simulink model "PV_Microgrid_700V_avg"  (R2025b)
settings: Solver=ode1  StartTime=0.0  StopTime=86400  FixedStep=10  RelTol=1e-3
settings Model: Creator=PC  LastModifiedBy=PC
settings DataIOCC: SaveOutput=off

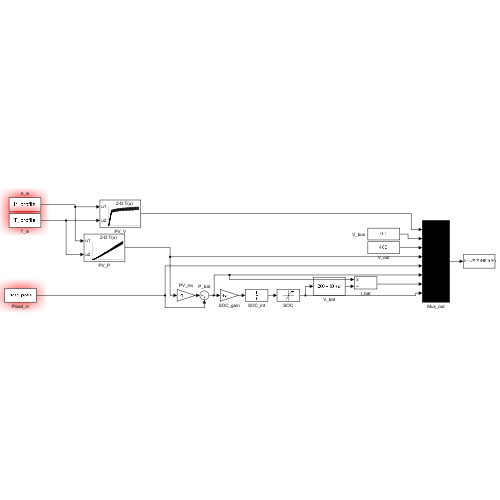
[thumbnail: Simulink's stored preview of the top-level diagram]
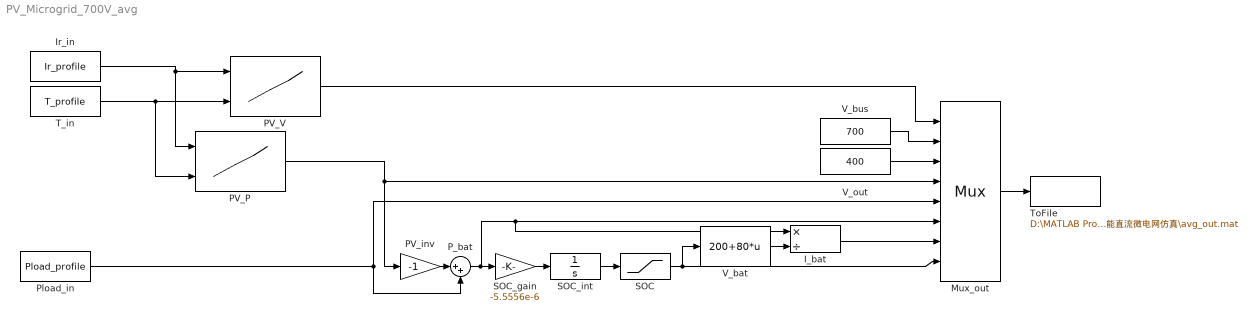
== system PV_Microgrid_700V_avg ==
  I_bat : Product  Inputs=*/
  Ir_in : FromWorkspace  VariableName=Ir_profile
  Mux_out : Mux  Inputs=8
  PV_P : Lookup_n-D  BreakpointsForDimension1=[0 100 200 300 400 500 600 700 800 900 1000]  BreakpointsForDimension2=[0 5 10 15 20 25 30 35 40 45]  Table=[0 0 0 0 0 0 0 0 0 0;479.267095176164 488.039274912844 496.8285763303 505.608509088825 514.379424979519 523.141658967104 531.90233605034 540.692996371929 549.47501520693 558.248690944814;1018.21000734054 1036.85645891559 1055.5023280483 1074.14764364788 1092.79243274262 1111.43672063028 1130.08053101432 1148.72388612752 1167.3668068442 1186.0093127824;1579.87273292352 1608.8143235643 1637.75152510228 1666.6845890358 1695.61374804727 1724.5392177273 1753.46119811304 1782.37987506345 1811.29542149157 1840.20799847052;2156.32163170459 2195.74523582645 2235.22493461024 2274.75056667442 2314.25580095053 2353.74186007896 2393.20987150242 2432.66087650542 2472.0958382476 2511.53595844375;2743.78589342684 2793.95276398475 2844.12262758078 2894.4417589686 2944.71315643147 2994.93984938429 3045.12461881785 3095.27002203532 3145.56779511549 3195.84887401155;3339.80841763825 3401.0911647803 3462.29044403554 3523.40716510524 3584.44687504203 3645.63503632356 3706.85652888916 3767.9997110104 3829.06951767878 3890.17475168714;3943.29173429922 4015.63363707419 4087.88520702704 4160.00939463728 4232.09113239226 4304.43299619547 4376.64909213525 4448.74777953302 4520.91939000649 4593.22084659552;4553.2053983687 4636.35277435902 4719.91035209304 4803.3036431147 4886.5208951813 4969.9265274586 5053.37839561389 5136.65963703153 5219.92730243945 5303.43282420516;5168.34686101416 5263.06947489515 5357.54448836249 5452.19614061513 5546.92870552013 5641.42542216233 5736.04537858514 5830.78693606171 5925.30333515889 6019.89458080095;5788.50808270469 5894.26936043688 6000.38379566756 6106.41353464746 6212.14007287575 6318.33198029437 6424.31326681351 6530.04226172463 6636.27038133268 6742.20810452584]  InternalRulePriority=Speed  RndMeth=Simplest
      settings: InputPortMap=u0,u1
  PV_V : Lookup_n-D  BreakpointsForDimension1=[0 100 200 300 400 500 600 700 800 900 1000]  BreakpointsForDimension2=[0 5 10 15 20 25 30 35 40 45]  Table=[0 0 0 0 0 0 0 0 0 0;308 312 318 324 330 336 340 346 352 358;324 330 336 342 348 354 360 366 372 378;336 342 348 354 360 366 372 378 384 390;342 348 356 362 368 374 380 386 392 400;348 354 362 368 374 380 386 392 400 406;352 360 366 372 378 386 392 398 404 412;356 364 370 376 384 390 396 402 410 416;360 366 374 380 386 394 400 406 414 420;364 370 376 384 390 396 404 410 416 424;366 372 380 386 392 400 406 414 420 426]  InternalRulePriority=Speed  RndMeth=Simplest
      settings: InputPortMap=u0,u1
  PV_inv : Gain  Gain=-1
  P_bat : Sum  Inputs=|++
  Pload_in : FromWorkspace  VariableName=Pload_profile
  SOC : Saturate  UpperLimit=0.9  LowerLimit=0.1
  SOC_gain : Gain  Gain=-5.5556e-6
  SOC_int : Integrator  InitialCondition=0.5
  T_in : FromWorkspace  VariableName=T_profile
  ToFile : ToFile  Filename=D:\MATLAB Project\Simulink\光伏储能直流微电网仿真\avg_out.mat  MatrixName=avgout  SaveFormat=Timeseries  SampleTime=60
  V_bat : Fcn  Expr=200+80*u
  V_bus : Constant  Value=700
  V_out : Constant  Value=400
  wires:
  Ir_in/1 -> PV_V/1, PV_P/1
  T_in/1 -> PV_V/2, PV_P/2
  Pload_in/1 -> P_bat/2, Mux_out/5
  PV_P/1 -> Mux_out/4, PV_inv/1
  PV_inv/1 -> P_bat/1
  P_bat/1 -> Mux_out/6, I_bat/1, SOC_gain/1
  SOC_gain/1 -> SOC_int/1
  SOC_int/1 -> SOC/1
  SOC/1 -> V_bat/1, Mux_out/8
  V_bat/1 -> I_bat/2
  PV_V/1 -> Mux_out/1
  V_bus/1 -> Mux_out/2
  V_out/1 -> Mux_out/3
  I_bat/1 -> Mux_out/7
  Mux_out/1 -> ToFile/1
